simulink model "example_hunt_crossley_bouncing_ball"  (Simulink 8.5)
settings: Solver=ode4  StartTime=0.0  StopTime=6  FixedStep=1e-5  RelTol=1e-3
InitFcn:
  | M =1;
  | 
  | R = 100e-3;
  | h=2*(1-0.334^2)/69e9;
  | h=h*1e3;
  | alpha=5000;
settings Model: Creator=toedtheide  LastModifiedBy=toedtheide
settings DataIOCC: SignalLoggingSaveFormat=Dataset
settings OptimizationCC: ExpressionDepthLimit=128
settings DebuggingCC: UnderspecifiedInitializationDetection=Simplified  MergeDetectMultiDrivingBlocksExec=error  FcnCallInpInsideContextMsg=EnableAllAsError  StateNameClashWarn=none
settings GRTTargetCC: CombineOutputUpdateFcns=on  GRTInterface=off

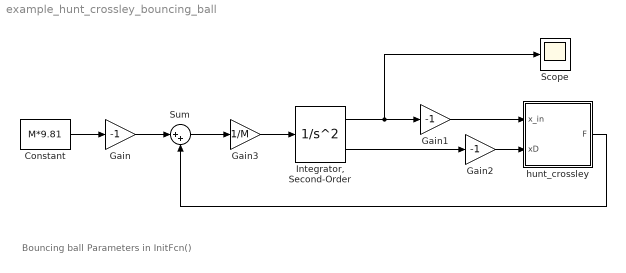
== system example_hunt_crossley_bouncing_ball ==
  note: Bouncing ball
      | Parameters in InitFcn()
  Constant : Constant  Value=M*9.81
  Gain : Gain  Gain=-1
  Gain1 : Gain  Gain=-1
  Gain2 : Gain  Gain=-1
  Gain3 : Gain  Gain=1/M
  "Integrator, Second-Order" : SecondOrderIntegrator  ICX=1  ICDXDT=0
  Scope : Scope
      settings: YMin=-0.05  YMax=1
  Sum : Sum  Inputs=|++
  hunt_crossley : MATLAB Function  TreatAsAtomicUnit=on
  wires:
  "Integrator, Second-Order"/1 -> Scope/1, Gain1/1
  "Integrator, Second-Order"/2 -> Gain2/1
  Gain1/1 -> hunt_crossley/1(x_in)
  Gain2/1 -> hunt_crossley/2(xD)
  Constant/1 -> Gain/1
  Gain/1 -> Sum/1
  hunt_crossley/1(F) -> Sum/2
  Sum/1 -> Gain3/1
  Gain3/1 -> "Integrator, Second-Order"/1

== matlab function hunt_crossley ==
  data: x_in input double; F output double; xD input double; R parameter double; h parameter double; alpha parameter double
function F = fcn(x_in, xD, R, h, alpha)
% Bouncing ball example
% Alexander Tödtheide, Institut für Regelungstechnik - 09-2016

if x_in > 0
  x = x_in;
else
  x = 0;
end

 [F_s,F_d]=Hunt_Crossley_contact_model_func(x,xD,R,h,alpha);

F = F_s + F_d;

end
